simulink model "PLL_Sim_Rev0"  (R2019b)
settings: Solver=VariableStepAuto  StartTime=0.0  StopTime=0.00002  RelTol=1e-3
libraries: impairlib x2
settings Model: Creator=connerhannon  LastModifiedBy=connerhannon

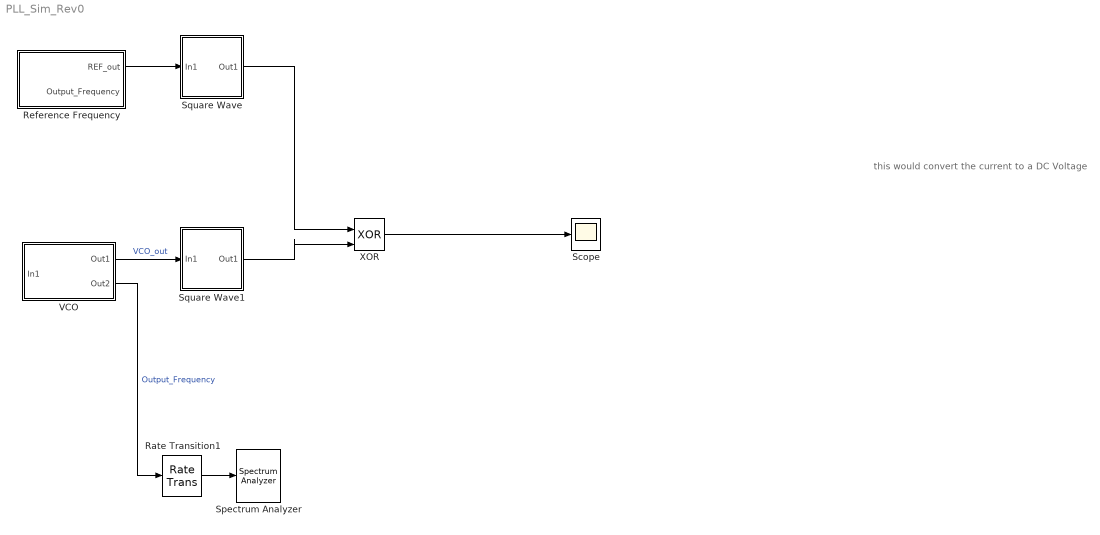
== system PLL_Sim_Rev0 ==
  note: this would convert the current to a DC Voltage
  Rate Transition1 : RateTransition  OutPortSampleTime=1e-9
  Reference Frequency : Subsystem
  Scope : Scope
  Spectrum Analyzer : SpectrumAnalyzer
  Square Wave : Subsystem
  Square Wave1 : Subsystem
  VCO : Subsystem
  XOR : Logic  Operator=XOR  IconShape=distinctive  AllPortsSameDT=off
  wires:
  XOR/1 -> Scope/1
  VCO/1(Out1) -> Square Wave1/1(In1)  "VCO_out"
  Rate Transition1/1 -> Spectrum Analyzer/1
  Reference Frequency/1(REF_out) -> Square Wave/1(In1)
  Square Wave/1(Out1) -> XOR/1
  Square Wave1/1(Out1) -> XOR/2
  VCO/2(Out2) -> Rate Transition1/1  "Output_Frequency"

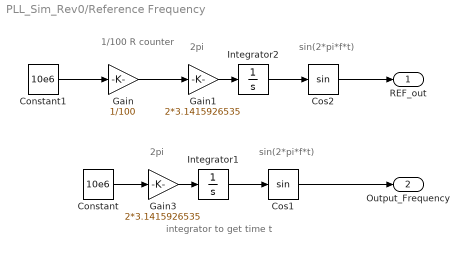
== system PLL_Sim_Rev0/Reference Frequency ==
  note: 1/100
      | R counter
  note: integrator to get time t
  note: sin(2*pi*f*t)
  note: 2pi
  note: sin(2*pi*f*t)
  note: 2pi
  Constant : Constant  Value=10e6
  Constant1 : Constant  Value=10e6
  Cos1 : Trigonometry  OutputSignalType=real
  Cos2 : Trigonometry  OutputSignalType=real
  Gain : Gain  Gain=1/100
  Gain1 : Gain  Gain=2*3.1415926535
  Gain3 : Gain  Gain=2*3.1415926535
  Integrator1 : Integrator
  Integrator2 : Integrator
  REF_out : Outport
  "Output_Frequency " : Outport  Port=2
  wires:
  Cos1/1 -> "Output_Frequency "/1
  Gain3/1 -> Integrator1/1
  Integrator1/1 -> Cos1/1
  Constant/1 -> Gain3/1
  Constant1/1 -> Gain/1
  Gain1/1 -> Integrator2/1
  Integrator2/1 -> Cos2/1
  Gain/1 -> Gain1/1
  Cos2/1 -> REF_out/1

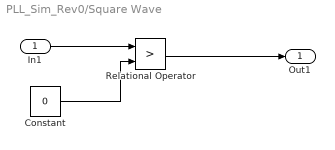
== system PLL_Sim_Rev0/Square Wave ==
  In1 : Inport
  Constant : Constant  Value=0
  Relational Operator : RelationalOperator  Operator=>  RndMeth=Nearest  InputSameDT=on
  Out1 : Outport
  wires:
  In1/1 -> Relational Operator/1
  Constant/1 -> Relational Operator/2
  Relational Operator/1 -> Out1/1

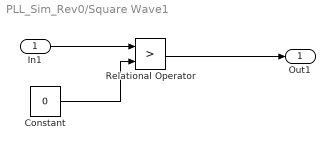
== system PLL_Sim_Rev0/Square Wave1 ==
  In1 : Inport
  Constant : Constant  Value=0
  Relational Operator : RelationalOperator  Operator=>  RndMeth=Nearest  InputSameDT=on
  Out1 : Outport
  wires:
  In1/1 -> Relational Operator/1
  Constant/1 -> Relational Operator/2
  Relational Operator/1 -> Out1/1

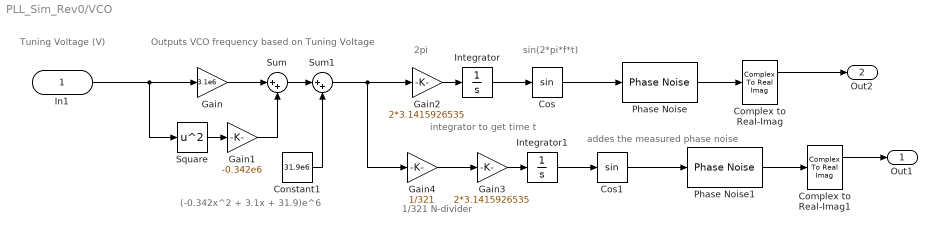
== system PLL_Sim_Rev0/VCO ==
  note: 1/321
      | N-divider
  note: Tuning Voltage
      | (V)
  note: 2pi
  note: sin(2*pi*f*t)
  note: integrator to get time t
  note: (-0.342x^2 + 3.1x + 31.9)e^6
  note: addes the measured phase noise
  note: Outputs VCO frequency based on Tuning Voltage
  In1 : Inport
  Complex to Real-Imag : ComplexToRealImag
  Complex to Real-Imag1 : ComplexToRealImag
  Constant1 : Constant  Value=31.9e6
  Cos : Trigonometry  OutputSignalType=complex
  Cos1 : Trigonometry  OutputSignalType=complex
  Gain : Gain  Gain=3.1e6
  Gain1 : Gain  Gain=-0.342e6
  Gain2 : Gain  Gain=2*3.1415926535
  Gain3 : Gain  Gain=2*3.1415926535
  Gain4 : Gain  Gain=1/321
  Integrator : Integrator
  Integrator1 : Integrator
  Phase Noise : impairlib/Phase Noise  Level=[ -36, -73, -83, -90, -112 ]  FrequencyOffset=[ 100, 400, 1000, 5000, 250000]  SampleRate=550000  RandomStream=mt19937ar with seed  Seed=1e6  SimulateUsing=Interpreted execution
      settings: SourceProductName=SerDes Toolbox  SourceProductBaseCode=SX
  Phase Noise1 : impairlib/Phase Noise  Level=[ -36, -73, -83, -90, -112 ]  FrequencyOffset=[ 100, 400, 1000, 5000, 250000]  SampleRate=550000  RandomStream=mt19937ar with seed  Seed=1e6  SimulateUsing=Interpreted execution
      settings: SourceProductName=SerDes Toolbox  SourceProductBaseCode=SX
  Square : Math  Operator=square  SignedPower=off  SaturateOnIntegerOverflow=on
  Sum : Sum  Inputs=|++
  Sum1 : Sum  Inputs=|++
  Out1 : Outport
  Out2 : Outport  Port=2
  wires:
  Gain1/1 -> Sum/2
  Gain/1 -> Sum/1
  Square/1 -> Gain1/1
  Integrator/1 -> Cos/1
  Constant1/1 -> Sum1/2
  Phase Noise/1 -> Complex to Real-Imag/1
  Sum1/1 -> Gain4/1, Gain2/1
  Sum/1 -> Sum1/1
  Cos/1 -> Phase Noise/1
  In1/1 -> Square/1, Gain/1
  Gain2/1 -> Integrator/1
  Gain3/1 -> Integrator1/1
  Phase Noise1/1 -> Complex to Real-Imag1/1
  Gain4/1 -> Gain3/1
  Cos1/1 -> Phase Noise1/1
  Integrator1/1 -> Cos1/1
  Complex to Real-Imag1/1 -> Out1/1
  Complex to Real-Imag/1 -> Out2/1
